simulink model "Close_loop_model"  (R2021a)
settings: Solver=VariableStepAuto  StartTime=0.0  StopTime=10.0  RelTol=1e-3
settings Model: Creator=ZYT  LastModifiedBy=ZYT

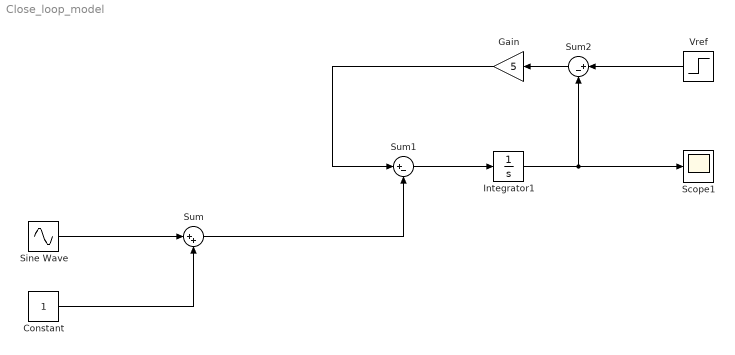
== system Close_loop_model ==
  Constant : Constant
  Gain : Gain  Gain=5
  Integrator1 : Integrator
  Scope1 : Scope
  Sine Wave : Sin  SampleTime=0
  Sum : Sum  Inputs=|++
  Sum1 : Sum  Inputs=|+-
  Sum2 : Sum  Inputs=|+-
  Vref : Step  SampleTime=0
  wires:
  Constant/1 -> Sum/2
  Sine Wave/1 -> Sum/1
  Sum/1 -> Sum1/2
  Sum1/1 -> Integrator1/1
  Integrator1/1 -> Sum2/2, Scope1/1
  Vref/1 -> Sum2/1
  Sum2/1 -> Gain/1
  Gain/1 -> Sum1/1
